simulink model "ball_bahn1"  (Simulink 4.00)
settings: Solver=ode45  StartTime=0.0  StopTime=20.0  RelTol=1e-3
settings Model: LastModifiedBy=Administrator  Refine=3  BlockReductionOpt=off

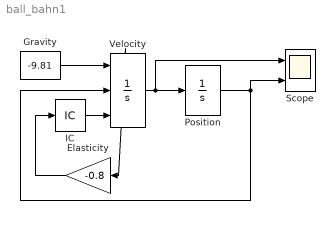
== system ball_bahn1 ==
  Elasticity : Gain  Orientation=left  Gain=-0.8  Multiplication=Element-wise(K.*u)  SaturateOnIntegerOverflow=on
  Gravity : Constant  Value=-9.81
  IC : InitialCondition  Value=15
  Position : Integrator  ExternalReset=none  InitialConditionSource=internal  InitialCondition=10  LimitOutput=on  UpperSaturationLimit=inf  LowerSaturationLimit=0  ShowSaturationPort=off  ShowStatePort=off  AbsoluteTolerance=auto
  Scope : Scope  NumInputPorts=2
      settings: TickLabels=on  TimeRange=auto  YMin=-30~0  YMax=20~22.9822  SaveToWorkspace=off  SaveName=ScopeData  DataFormat=Array  LimitDataPoints=on  MaxDataPoints=5000
  Velocity : Integrator  ExternalReset=falling  InitialConditionSource=external  InitialCondition=0  LimitOutput=off  UpperSaturationLimit=inf  LowerSaturationLimit=-inf  ShowSaturationPort=off  ShowStatePort=on  AbsoluteTolerance=auto
  wires:
  Velocity/State -> Elasticity/1
  IC/1 -> Velocity/3
  Elasticity/1 -> IC/1
  Velocity/1 -> Position/1, Scope/1
  Position/1 -> Scope/2, Velocity/2
  Gravity/1 -> Velocity/1
